simulink model "Controller1_2"  (R2018b)
settings: Solver=ode3  StartTime=0.0  StopTime=inf  FixedStep=Ts  RelTol=1e-3
InitFcn:
  | Ts=0.015; %采样时间
  | R=0.0344 %车轮半径，m
  | Wr=290 %赛道宽度290mm
  | Wc=187 %小车宽度187mm
  | Wl=250; %限宽门宽度250mm
  | K1=[0.4175;0.5498]; %速度控制的Ki、Kp参数
  | K2=[0.02;0.7]; %转向控制的Kd、Kp参数
undefined symbols (not defined in the file): DiscIntNeverNeededParam
libraries: simulink x6, legoev3lib x5, simulink_extras x1
settings Model: SimulationMode=external  ExtModeTrigDuration=2  Creator=The MathWorks, Inc.  LastModifiedBy=adminstrator
settings SolverCC: PositivePriorityOrder=on
settings DataIOCC: LimitDataPoints=on  SaveFormat=Array
settings OptimizationCC: LifeSpan=Inf  MaxStackSize=64
settings DebuggingCC: UnderspecifiedInitializationDetection=Classic  MergeDetectMultiDrivingBlocksExec=none  AllowSymbolicDim=off  SFUnexpectedBacktrackingDiag=warning  SFNoUnconditionalDefaultTransitionDiag=warning  SFExecutionAtInitializationDiag=none
settings HardwareCC: ProdBitPerPointer=32  ProdBitPerSizeT=32  ProdBitPerPtrDiffT=32  ProdLargestAtomicInteger=Long  ProdWordSize=32  ProdHWDeviceType=ARM Compatible->ARM 9  TargetLargestAtomicInteger=Long  TargetLargestAtomicFloat=Float  TargetIntDivRoundTo=Zero  TargetEndianess=LittleEndian  TargetHWDeviceType=ARM Compatible->ARM 9
settings ModelReferenceCC: PropagateSignalLabelsOutOfModel=off
settings SFSimCC: SimUseLocalCustomCode=off  SimGenImportedTypeDefs=on
settings RTWCC: SystemTargetFile=ert.tlc  HardwareBoard=LEGO MINDSTORMS EV3  TemplateMakefile=ert_default_tmf  GenerateReport=on  RTWVerbose=off  RTWUseLocalCustomCode=off  Toolchain=Sourcery G++ Lite v2009q3  BuildConfiguration=Faster Runs  LaunchReport=on
settings CodeAppCC: ForceParamTrailComments=on  OperatorAnnotations=on  StateflowObjectComments=on  MATLABSourceComments=on
settings ERTTargetCC: MultiwordLength=2048  ERTCustomFileBanners=off  SupportContinuousTime=on  SupportNonInlinedSFcns=on  RemoveResetFunc=off  ModelStepFunctionPrototypeControlCompliant=off
settings ConfigComp: CovMetricSettings=dw  CovHtmlReporting=on  CovSaveCumulativeToWorkspaceVar=on  CovSaveSingleToWorkspaceVar=on  CovExternalEMLEnable=off  CovSFcnEnable=off

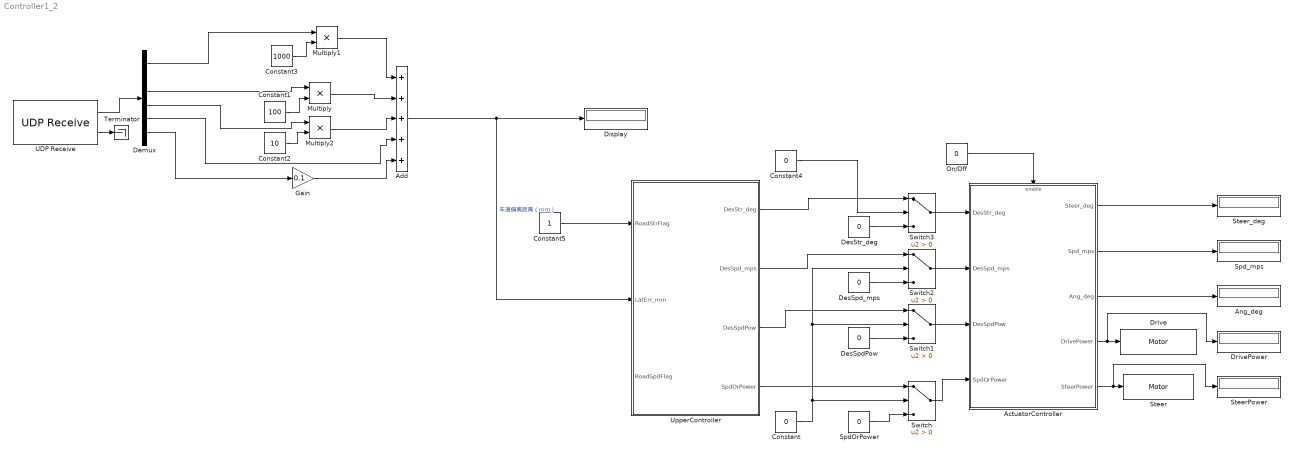
== system Controller1_2 ==
  ActuatorController : Subsystem
  Add : Sum  Inputs=+++++
  Ang_deg : Display
  Constant : Constant  Value=0
  Constant1 : Constant  Value=100
  Constant2 : Constant  Value=10
  Constant3 : Constant  Value=1000
  Constant4 : Constant  Value=0
  Constant5 : Constant
  Demux : Demux  Outputs=6
  DesSpdPow : Constant  Value=0
  DesSpd_mps : Constant  Value=0
  DesStr_deg : Constant  Value=0
  Display : Display
  Drive : legoev3lib/Motor  sportNumber=A  sstopAction=Brake
  DrivePower : Display
  Gain : Gain  Gain=0.1
  Multiply : Product
  Multiply1 : Product
  Multiply2 : Product
  On/Off : Constant  Value=0
  SpdOrPower : Constant  Value=0
  Spd_mps : Display
  Steer : legoev3lib/Motor  sportNumber=B  sstopAction=Brake
  SteerPower : Display
  Steer_deg : Display
  Switch{,1..3} (4 alike) : Switch  Criteria=u2 > Threshold
  Terminator : Terminator
  UDP Receive : legoev3lib/UDP Receive  localURL='0.0.0.0'  localPort=25000  remoteURL='0.0.0.0'  remotePort=-1  recvBufferSize=8192  signalDatatype=uint8  dims=6  isVarSize=off  showBlockingTime=off  blockingTime=0  sampletime=Ts  blockPlatform=LEGO EV3
      settings: SourceProductName=Simulink Support Package for LEGO MINDSTORMS EV3 Hardware  SourceProductBaseCode=LEGOEV3
  UpperController : Subsystem
  wires:
  On/Off/1 -> ActuatorController/Enable
  Switch/1 -> ActuatorController/4(SpdOrPower)
  Constant/1 -> Switch2/2, Switch1/2, Switch/2
  SpdOrPower/1 -> Switch/3
  DesSpdPow/1 -> Switch1/3
  Switch1/1 -> ActuatorController/3(DesSpdPow)
  Switch2/1 -> ActuatorController/2(DesSpd_mps)
  UpperController/2(DesSpd_mps) -> Switch2/1
  DesSpd_mps/1 -> Switch2/3
  Switch3/1 -> ActuatorController/1(DesStr_deg)
  Constant4/1 -> Switch3/2
  DesStr_deg/1 -> Switch3/3
  ActuatorController/5(SteerPower) -> Steer/1, SteerPower/1
  ActuatorController/1(Steer_deg) -> Steer_deg/1
  ActuatorController/2(Spd_mps) -> Spd_mps/1
  ActuatorController/3(Ang_deg) -> Ang_deg/1
  ActuatorController/4(DrivePower) -> Drive/1, DrivePower/1
  UpperController/3(DesSpdPow) -> Switch1/1
  UpperController/1(DesStr_deg) -> Switch3/1
  UpperController/4(SpdOrPower) -> Switch/1
  Demux/3 -> Multiply/1
  Constant2/1 -> Multiply2/2
  Demux/5 -> Add/4
  Multiply2/1 -> Add/3
  Multiply/1 -> Add/2
  Demux/4 -> Multiply2/1
  Add/1 -> Display/1, UpperController/2(LatErr_mm)  "车道偏离距离（mm）"
  Constant1/1 -> Multiply/2
  UDP Receive/1 -> Demux/1
  Constant3/1 -> Multiply1/2
  Multiply1/1 -> Add/1
  Demux/1 -> Multiply1/1
  UDP Receive/2 -> Terminator/1
  Constant5/1 -> UpperController/1(RoadStrFlag)
  Demux/6 -> Gain/1
  Gain/1 -> Add/5

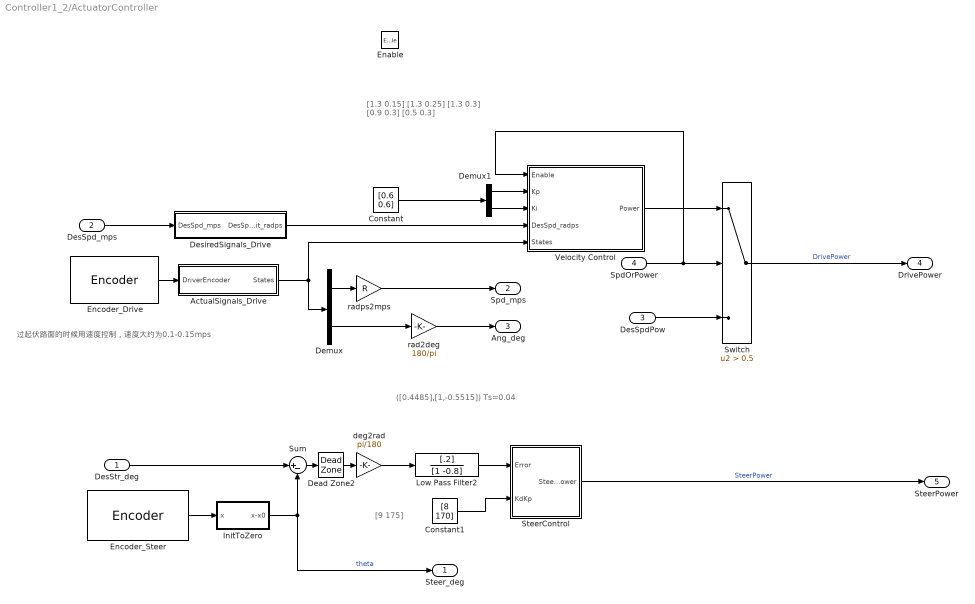
== system Controller1_2/ActuatorController ==
  note: ([0.4485],[1,-0.5515]) Ts=0.04
  note: [9 175]
  note: [1.3 0.15]
      | [1.3 0.25]
      | [1.3 0.3]
      | [0.9 0.3]
      | [0.5 0.3]
  note: 过起伏路面的时候用速度控制，速度大约为0.1-0.15mps
  DesStr_deg : Inport
  DesSpd_mps : Inport  Port=2
  DesSpdPow : Inport  Port=3
  SpdOrPower : Inport  Port=4
  Enable : EnablePort  StatesWhenEnabling=reset
  ActualSignals_Drive : Subsystem
  Constant : Constant  Value=[0.6 0.6]
  Constant1 : Constant  Value=[8 170]
  Dead Zone2 : DeadZone  LowerValue=-1  UpperValue=1  SaturateOnIntegerOverflow=on
  Demux : Demux  Outputs=2
  Demux1 : Demux  Outputs=2
  DesiredSignals_Drive : Subsystem
  Encoder_Drive : legoev3lib/Encoder  portNumber=A  opMode=No reset  sampleTime=Ts
      settings: SourceProductName=Simulink Support Package for LEGO MINDSTORMS EV3 Hardware  SourceProductBaseCode=LEGOEV3
  Encoder_Steer : legoev3lib/Encoder  portNumber=B  opMode=No reset  sampleTime=Ts
      settings: SourceProductName=Simulink Support Package for LEGO MINDSTORMS EV3 Hardware  SourceProductBaseCode=LEGOEV3
  InitToZero : Subsystem
  Low Pass Filter2 : DiscreteFilter  Numerator=[.2]  Denominator=[1 -0.8]
  SteerControl : Subsystem
  Sum : Sum  Inputs=|+-
  Switch : Switch  Criteria=u2 > Threshold  Threshold=0.5
  Velocity Control : Subsystem
  deg2rad : Gain  Gain=pi/180
  rad2deg : Gain  Gain=180/pi
  radps2mps : Gain  Gain=R
  Steer_deg : Outport
  Spd_mps : Outport  Port=2
  Ang_deg : Outport  Port=3
  DrivePower : Outport  Port=4  OutputWhenDisabled=reset  InitialOutput=0
  SteerPower : Outport  Port=5  OutputWhenDisabled=reset  InitialOutput=0
  wires:
  deg2rad/1 -> Low Pass Filter2/1
  Demux1/1 -> Velocity Control/2(Kp)
  Demux/2 -> rad2deg/1
  DesiredSignals_Drive/1(DesSpdFit_radps) -> Velocity Control/4(DesSpd_radps)
  Dead Zone2/1 -> deg2rad/1
  radps2mps/1 -> Spd_mps/1
  rad2deg/1 -> Ang_deg/1
  Demux1/2 -> Velocity Control/3(Ki)
  Constant1/1 -> SteerControl/2(KdKp)
  InitToZero/1(x-x0) -> Steer_deg/1, Sum/2  "theta"
  ActualSignals_Drive/1("States ") -> Demux/1, Velocity Control/5(States)
  SpdOrPower/1 -> Switch/2, Velocity Control/1("Enable ")
  DesStr_deg/1 -> Sum/1
  Constant/1 -> Demux1/1
  Sum/1 -> Dead Zone2/1
  Encoder_Drive/1 -> ActualSignals_Drive/1(DriverEncoder)
  Velocity Control/1(Power) -> Switch/1
  Demux/1 -> radps2mps/1
  DesSpd_mps/1 -> DesiredSignals_Drive/1(DesSpd_mps)
  Encoder_Steer/1 -> InitToZero/1(x)
  Low Pass Filter2/1 -> SteerControl/1(Error)
  Switch/1 -> DrivePower/1  "DrivePower"
  SteerControl/1(SteerPower) -> SteerPower/1  "SteerPower"
  DesSpdPow/1 -> Switch/3

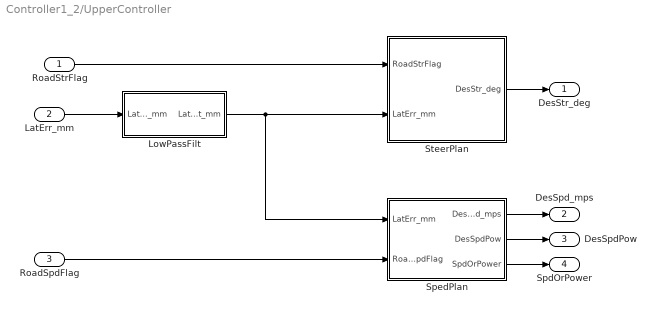
== system Controller1_2/UpperController ==
  RoadStrFlag : Inport
  LatErr_mm : Inport  Port=2
  RoadSpdFlag : Inport  Port=3
  LowPassFilt : Subsystem
  SpedPlan : Subsystem
  SteerPlan : Subsystem
  DesStr_deg : Outport
  DesSpd_mps : Outport  Port=2
  DesSpdPow : Outport  Port=3
  SpdOrPower : Outport  Port=4
  wires:
  LatErr_mm/1 -> LowPassFilt/1(LatErr_mm)
  LowPassFilt/1(LatErrFit_mm) -> SpedPlan/1(LatErr_mm), SteerPlan/2(LatErr_mm)
  SteerPlan/1(DesStr_deg) -> DesStr_deg/1
  SpedPlan/1(DesSpd_mps) -> DesSpd_mps/1
  SpedPlan/2(DesSpdPow) -> DesSpdPow/1
  SpedPlan/3(SpdOrPower) -> SpdOrPower/1
  RoadSpdFlag/1 -> SpedPlan/2(RoadSpdFlag)
  RoadStrFlag/1 -> SteerPlan/1(RoadStrFlag)

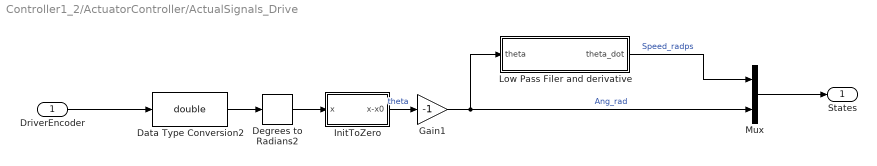
== system Controller1_2/ActuatorController/ActualSignals_Drive ==
  DriverEncoder : Inport
  Data Type Conversion2 : DataTypeConversion  OutDataTypeStr=double
  Degrees to Radians2 : simulink_extras/Transformations/Degrees to Radians
  Gain1 : Gain  Gain=-1
  InitToZero : Subsystem
  Low Pass Filer and derivative : Subsystem
  Mux : Mux  Inputs=2
  "States " : Outport
  wires:
  Degrees to Radians2/1 -> InitToZero/1(x)
  Data Type Conversion2/1 -> Degrees to Radians2/1
  InitToZero/1(x-x0) -> Gain1/1  "theta"
  DriverEncoder/1 -> Data Type Conversion2/1
  Gain1/1 -> Low Pass Filer and derivative/1(theta), Mux/2  "Ang_rad"
  Mux/1 -> "States "/1
  Low Pass Filer and derivative/1(theta_dot) -> Mux/1  "Speed_radps"

== system Controller1_2/ActuatorController/DesiredSignals_Drive ==
  DesSpd_mps : Inport
  Low Pass Filter2 : DiscreteFilter  Numerator=[0.15]  Denominator=[1 -0.85]
  m/s --> rad/s : Gain  Gain=1/R
  DesSpdFit_radps : Outport
  wires:
  m/s --> rad/s/1 -> Low Pass Filter2/1  "des_theta_dot"
  DesSpd_mps/1 -> m/s --> rad/s/1
  Low Pass Filter2/1 -> DesSpdFit_radps/1

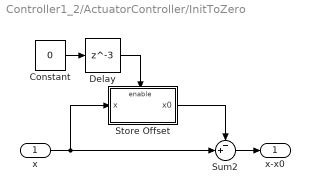
== system Controller1_2/ActuatorController/InitToZero ==
  x : Inport
  Constant : Constant  Value=0  OutDataTypeStr=boolean
  Delay : Delay  DelayLength=3  InitialCondition=1
  Store Offset : Subsystem  TreatAsAtomicUnit=on
  Sum2 : Sum  Inputs=-+|
  x-x0 : Outport
  wires:
  x/1 -> Sum2/2, Store Offset/1(x)
  Store Offset/1(x0) -> Sum2/1
  Constant/1 -> Delay/1
  Delay/1 -> Store Offset/Enable
  Sum2/1 -> x-x0/1

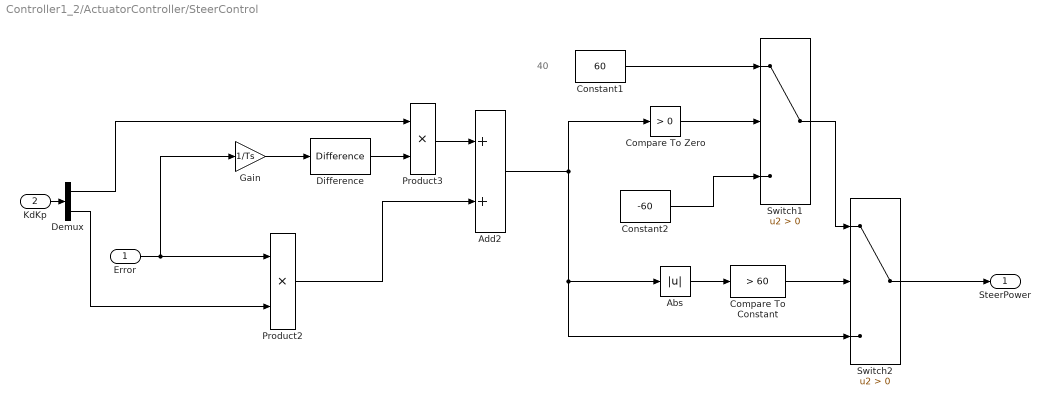
== system Controller1_2/ActuatorController/SteerControl ==
  note: 40
  Error : Inport
  KdKp : Inport  Port=2
  Abs : Abs
  Add2 : Sum
  Compare To Constant : simulink/Logic and Bit Operations/Compare To Constant  relop=>  const=60  OutDataTypeStr=boolean
  Compare To Zero : simulink/Logic and Bit Operations/Compare To Zero  relop=>  OutDataTypeStr=boolean
  Constant1 : Constant  Value=60
  Constant2 : Constant  Value=-60
  Demux : Demux  Outputs=2
  Difference : simulink/Discrete/Difference  ICPrevInput=0.0  OutMin=[]  OutMax=[]  OutDataType=fixdt(1, 16)  OutScaling=2^-10  DoSatur=off
  Gain : Gain  Gain=1/Ts
  Product2 : Product
  Product3 : Product
  Switch1 : Switch  Criteria=u2 > Threshold
  Switch2 : Switch  Criteria=u2 > Threshold
  SteerPower : Outport
  wires:
  Constant1/1 -> Switch1/1
  Switch2/1 -> SteerPower/1
  Demux/2 -> Product2/2
  Difference/1 -> Product3/2
  Add2/1 -> Compare To Zero/1, Switch2/3, Abs/1
  Product2/1 -> Add2/2
  Compare To Constant/1 -> Switch2/2
  Demux/1 -> Product3/1
  Product3/1 -> Add2/1
  Compare To Zero/1 -> Switch1/2
  Constant2/1 -> Switch1/3
  Switch1/1 -> Switch2/1
  Abs/1 -> Compare To Constant/1
  Error/1 -> Gain/1, Product2/1
  Gain/1 -> Difference/1
  KdKp/1 -> Demux/1

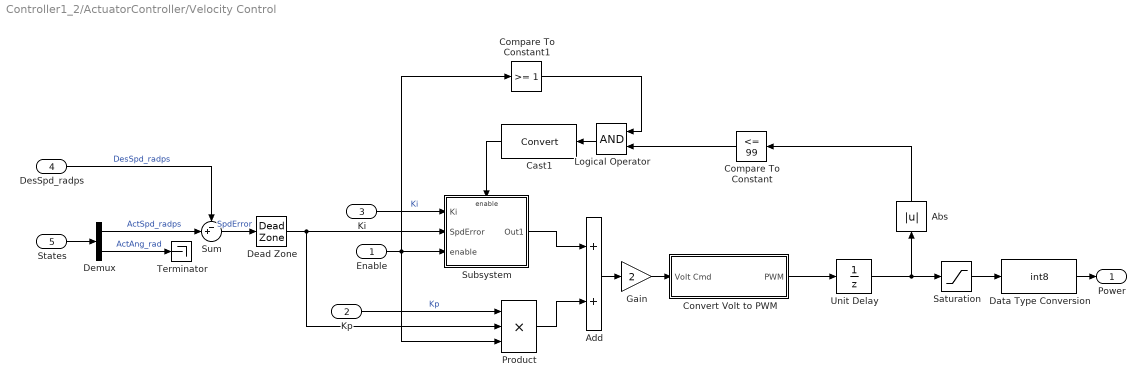
== system Controller1_2/ActuatorController/Velocity Control ==
  "Enable " : Inport
  Kp : Inport  Port=2
  Ki : Inport  Port=3
  DesSpd_radps : Inport  Port=4
  States : Inport  Port=5
  Abs : Abs
  Add : Sum
  Cast1 : DataTypeConversion
  Compare To Constant : simulink/Logic and Bit Operations/Compare To Constant  relop=<=  const=99  OutDataTypeStr=boolean
  Compare To Constant1 : simulink/Logic and Bit Operations/Compare To Constant  relop=>=  const=1  OutDataTypeStr=boolean
  Convert Volt to PWM : Subsystem
  Data Type Conversion : DataTypeConversion  OutDataTypeStr=int8
  Dead Zone : DeadZone  LowerValue=-0.01  UpperValue=0.01  SaturateOnIntegerOverflow=on
  Demux : Demux  Outputs=2
  Gain : Gain  Gain=2
  Logical Operator : Logic  AllPortsSameDT=off  OutDataTypeStr=boolean
  Product : Product  Inputs=3
  Saturation : Saturate  UpperLimit=100  LowerLimit=-100
  Subsystem : Subsystem
  Sum : Sum  Inputs=-+|
  Terminator : Terminator
  Unit Delay : UnitDelay  SampleTime=-1
  Power : Outport  OutputWhenDisabled=reset  InitialOutput=0
  wires:
  Add/1 -> Gain/1
  Gain/1 -> Convert Volt to PWM/1(Volt Cmd)
  DesSpd_radps/1 -> Sum/1  "DesSpd_radps"
  States/1 -> Demux/1
  Demux/1 -> Sum/2  "ActSpd_radps"
  Demux/2 -> Terminator/1  "ActAng_rad"
  Sum/1 -> Dead Zone/1  "SpdError"
  Ki/1 -> Subsystem/1(Ki)  "Ki"
  Product/1 -> Add/2
  Subsystem/1(Out1) -> Add/1
  Kp/1 -> Product/1  "Kp"
  Abs/1 -> Compare To Constant/1
  Compare To Constant/1 -> Logical Operator/2
  Data Type Conversion/1 -> Power/1
  Saturation/1 -> Data Type Conversion/1
  Compare To Constant1/1 -> Logical Operator/1
  Logical Operator/1 -> Cast1/1
  Cast1/1 -> Subsystem/Enable
  Convert Volt to PWM/1(PWM) -> Unit Delay/1
  "Enable "/1 -> Product/3, Compare To Constant1/1, Subsystem/3(enable)
  Unit Delay/1 -> Saturation/1, Abs/1
  Dead Zone/1 -> Product/2, Subsystem/2(SpdError)

== system Controller1_2/UpperController/LowPassFilt ==
  LatErr_mm : Inport
  Discrete Filter : DiscreteFilter  Numerator=[0.2 0.3669]  Denominator=[1 -0.4331]
  LatErrFit_mm : Outport
  wires:
  LatErr_mm/1 -> Discrete Filter/1
  Discrete Filter/1 -> LatErrFit_mm/1

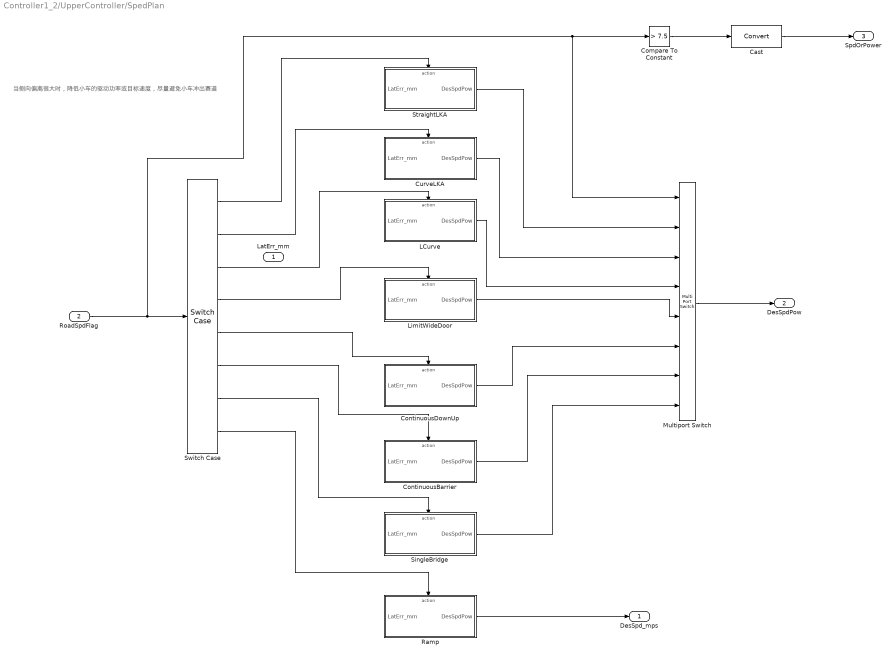
== system Controller1_2/UpperController/SpedPlan ==
  note: 当侧向偏离很大时，降低小车的驱动功率或目标速度，尽量避免小车冲出赛道
  LatErr_mm : Inport
  RoadSpdFlag : Inport  Port=2
  Cast : DataTypeConversion
  Compare To Constant : simulink/Logic and Bit Operations/Compare To Constant  relop=>  const=7.5  OutDataTypeStr=boolean
  ContinuousBarrier : Subsystem  TreatAsAtomicUnit=on
  ContinuousDownUp : Subsystem  TreatAsAtomicUnit=on
  CurveLKA : Subsystem  TreatAsAtomicUnit=on
  LCurve : Subsystem  TreatAsAtomicUnit=on
  LimitWideDoor : Subsystem  TreatAsAtomicUnit=on
  Multiport Switch : MultiPortSwitch  Inputs=7
  Ramp : Subsystem  TreatAsAtomicUnit=on
  SingleBridge : Subsystem  TreatAsAtomicUnit=on
  StraightLKA : Subsystem  TreatAsAtomicUnit=on
  Switch Case : SwitchCase  CaseConditions={1,2,3,4,5,6,7,8}  ShowDefaultCase=off
  DesSpd_mps : Outport
  DesSpdPow : Outport  Port=2
  SpdOrPower : Outport  Port=3
  wires:
  Switch Case/1 -> StraightLKA/Action
  Switch Case/2 -> CurveLKA/Action
  Switch Case/3 -> LCurve/Action
  Switch Case/4 -> LimitWideDoor/Action
  Switch Case/5 -> ContinuousDownUp/Action
  Switch Case/6 -> ContinuousBarrier/Action
  Switch Case/7 -> SingleBridge/Action
  Switch Case/8 -> Ramp/Action
  Multiport Switch/1 -> DesSpdPow/1
  RoadSpdFlag/1 -> Multiport Switch/1, Compare To Constant/1, Switch Case/1
  StraightLKA/1(DesSpdPow) -> Multiport Switch/2
  CurveLKA/1(DesSpdPow) -> Multiport Switch/3
  LCurve/1(DesSpdPow) -> Multiport Switch/4
  LimitWideDoor/1(DesSpdPow) -> Multiport Switch/5
  ContinuousDownUp/1(DesSpdPow) -> Multiport Switch/6
  ContinuousBarrier/1(DesSpdPow) -> Multiport Switch/7
  SingleBridge/1(DesSpdPow) -> Multiport Switch/8
  Ramp/1(DesSpdPow) -> DesSpd_mps/1
  Compare To Constant/1 -> Cast/1
  Cast/1 -> SpdOrPower/1

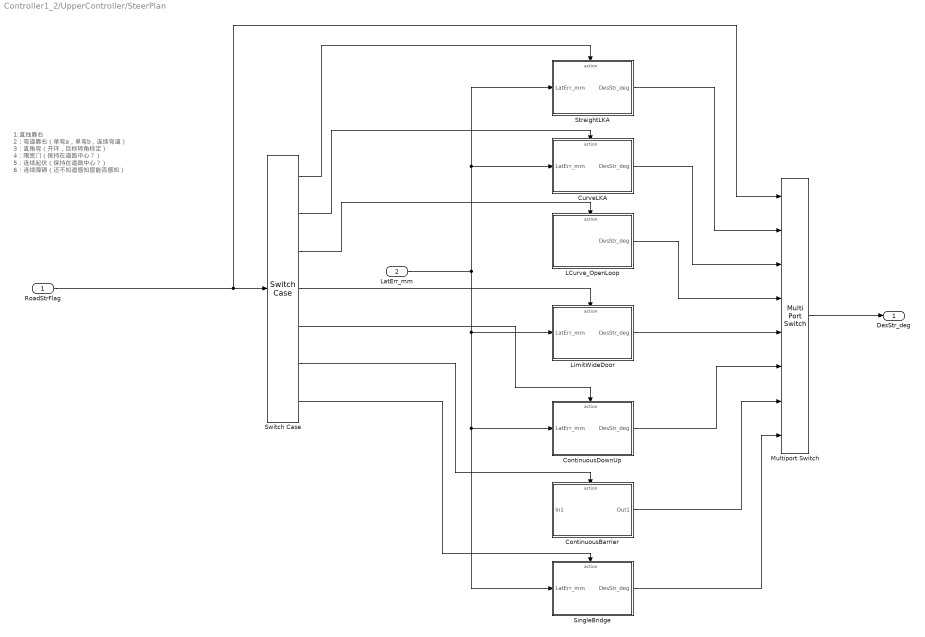
== system Controller1_2/UpperController/SteerPlan ==
  note: 1:直线靠右
      | 2：弯道靠右（单弯a，单弯b，连续弯道）
      | 3：直角弯（开环，目标转角标定）
      | 4：限宽门（保持在道路中心？）
      | 5：连续起伏（保持在道路中心？）
      | 6：连续障碍（还不知道感知层能否感知）
  RoadStrFlag : Inport
  LatErr_mm : Inport  Port=2
  ContinuousBarrier : Subsystem  TreatAsAtomicUnit=on
  ContinuousDownUp : Subsystem  TreatAsAtomicUnit=on
  CurveLKA : Subsystem  TreatAsAtomicUnit=on
  LCurve_OpenLoop : Subsystem  TreatAsAtomicUnit=on
  LimitWideDoor : Subsystem  TreatAsAtomicUnit=on
  Multiport Switch : MultiPortSwitch  Inputs=7
  SingleBridge : Subsystem  TreatAsAtomicUnit=on
  StraightLKA : Subsystem  TreatAsAtomicUnit=on
  Switch Case : SwitchCase  CaseConditions={1,2,3,4,5,6,7}  ShowDefaultCase=off
  DesStr_deg : Outport
  wires:
  RoadStrFlag/1 -> Multiport Switch/1, Switch Case/1
  Switch Case/2 -> CurveLKA/Action
  Switch Case/3 -> LCurve_OpenLoop/Action
  Switch Case/4 -> LimitWideDoor/Action
  Switch Case/5 -> ContinuousDownUp/Action
  Switch Case/6 -> ContinuousBarrier/Action
  Multiport Switch/1 -> DesStr_deg/1
  StraightLKA/1(DesStr_deg) -> Multiport Switch/2
  CurveLKA/1(DesStr_deg) -> Multiport Switch/3
  LCurve_OpenLoop/1(DesStr_deg) -> Multiport Switch/4
  LimitWideDoor/1(DesStr_deg) -> Multiport Switch/5
  ContinuousDownUp/1(DesStr_deg) -> Multiport Switch/6
  ContinuousBarrier/1(Out1) -> Multiport Switch/7
  LatErr_mm/1 -> CurveLKA/1(LatErr_mm), StraightLKA/1(LatErr_mm), LimitWideDoor/1(LatErr_mm), SingleBridge/1(LatErr_mm), ContinuousDownUp/1(LatErr_mm)
  Switch Case/7 -> SingleBridge/Action
  Switch Case/1 -> StraightLKA/Action
  SingleBridge/1(DesStr_deg) -> Multiport Switch/8

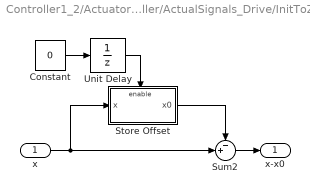
== system Controller1_2/ActuatorController/ActualSignals_Drive/InitToZero ==
  x : Inport
  Constant : Constant  Value=0  OutDataTypeStr=boolean
  Store Offset : Subsystem  TreatAsAtomicUnit=on
  Sum2 : Sum  Inputs=-+|
  Unit Delay : UnitDelay  InitialCondition=1  SampleTime=-1
  x-x0 : Outport
  wires:
  x/1 -> Sum2/2, Store Offset/1(x)
  Store Offset/1(x0) -> Sum2/1
  Constant/1 -> Unit Delay/1
  Unit Delay/1 -> Store Offset/Enable
  Sum2/1 -> x-x0/1

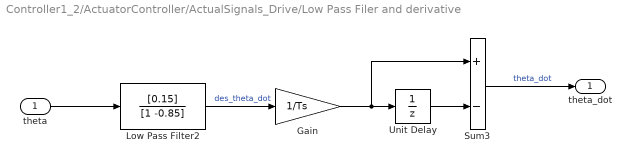
== system Controller1_2/ActuatorController/ActualSignals_Drive/Low Pass Filer and derivative ==
  theta : Inport
  Gain : Gain  Gain=1/Ts
  Low Pass Filter2 : DiscreteFilter  Numerator=[0.15]  Denominator=[1 -0.85]
  Sum3 : Sum  Inputs=+-
  Unit Delay : UnitDelay  SampleTime=-1
  theta_dot : Outport
  wires:
  theta/1 -> Low Pass Filter2/1
  Sum3/1 -> theta_dot/1  "theta_dot"
  Gain/1 -> Sum3/1, Unit Delay/1
  Unit Delay/1 -> Sum3/2
  Low Pass Filter2/1 -> Gain/1  "des_theta_dot"

== system Controller1_2/ActuatorController/InitToZero/Store Offset ==
  x : Inport
  Enable : EnablePort
  x0 : Outport  InitialOutput=0
  wires:
  x/1 -> x0/1

== system Controller1_2/ActuatorController/Velocity Control/Convert Volt to PWM ==
  note: Normalization by maximum voltage
      | and
      | Scaling to PWM
  Volt Cmd : Inport
  Battery Voltage : Subsystem
  Divide : Product  Inputs=*/
  Gain : Gain  Gain=100
  Low Pass Filter : DiscreteFilter  Numerator=[0.15]  Denominator=[1 -0.85]
  PWM : Outport
  wires:
  Battery Voltage/1(Battery) -> Divide/2
  Divide/1 -> Gain/1
  Volt Cmd/1 -> Low Pass Filter/1  "des_theta_dot"
  Gain/1 -> PWM/1
  Low Pass Filter/1 -> Divide/1

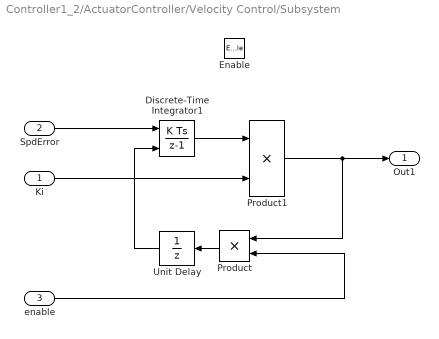
== system Controller1_2/ActuatorController/Velocity Control/Subsystem ==
  Ki : Inport
  SpdError : Inport  Port=2
  enable : Inport  Port=3
  Enable : EnablePort  StatesWhenEnabling=reset
  Discrete-Time Integrator1 : DiscreteIntegrator  InitialConditionSource=external  SampleTime=-1  ICPrevOutput=DiscIntNeverNeededParam  ICPrevScaledInput=DiscIntNeverNeededParam
  Product : Product
  Product1 : Product
  Unit Delay : UnitDelay  SampleTime=-1
  Out1 : Outport
  wires:
  Ki/1 -> Product1/2
  Discrete-Time Integrator1/1 -> Product1/1
  Product1/1 -> Product/1, Out1/1
  SpdError/1 -> Discrete-Time Integrator1/1
  enable/1 -> Product/2
  Product/1 -> Unit Delay/1
  Unit Delay/1 -> Discrete-Time Integrator1/2

== system Controller1_2/UpperController/SpedPlan/ContinuousBarrier ==
  LatErr_mm : Inport
  Action Port : ActionPort  ActionType=case
  DesSpdPow : Outport
  wires:
  LatErr_mm/1 -> DesSpdPow/1

== system Controller1_2/UpperController/SpedPlan/ContinuousDownUp ==
  LatErr_mm : Inport
  Action Port : ActionPort  ActionType=case
  DesSpdPow : Outport
  wires:
  LatErr_mm/1 -> DesSpdPow/1

== system Controller1_2/UpperController/SpedPlan/CurveLKA ==
  LatErr_mm : Inport
  Action Port : ActionPort  ActionType=case
  DesSpdPow : Outport
  wires:
  LatErr_mm/1 -> DesSpdPow/1

== system Controller1_2/UpperController/SpedPlan/LCurve ==
  LatErr_mm : Inport
  Action Port : ActionPort  ActionType=case
  DesSpdPow : Outport
  wires:
  LatErr_mm/1 -> DesSpdPow/1

== system Controller1_2/UpperController/SpedPlan/LimitWideDoor ==
  LatErr_mm : Inport
  Action Port : ActionPort  ActionType=case
  DesSpdPow : Outport
  wires:
  LatErr_mm/1 -> DesSpdPow/1

== system Controller1_2/UpperController/SpedPlan/Ramp ==
  LatErr_mm : Inport
  Action Port : ActionPort  ActionType=case
  DesSpdPow : Outport
  wires:
  LatErr_mm/1 -> DesSpdPow/1

== system Controller1_2/UpperController/SpedPlan/SingleBridge ==
  LatErr_mm : Inport
  Action Port : ActionPort  ActionType=case
  DesSpdPow : Outport
  wires:
  LatErr_mm/1 -> DesSpdPow/1

== system Controller1_2/UpperController/SpedPlan/StraightLKA ==
  LatErr_mm : Inport
  Action Port : ActionPort  ActionType=case
  DesSpdPow : Outport
  wires:
  LatErr_mm/1 -> DesSpdPow/1

== system Controller1_2/UpperController/SteerPlan/ContinuousBarrier ==
  In1 : Inport
  Action Port : ActionPort  ActionType=case
  Out1 : Outport
  wires:
  In1/1 -> Out1/1

== system Controller1_2/UpperController/SteerPlan/ContinuousDownUp ==
  note: 和直线车道保持一样，之所以和直线LKA分开，是考虑到后续调参的时候可能会和直线LKA不太一样
  LatErr_mm : Inport
  Action Port : ActionPort  ActionType=case
  Constant : Constant  Value=Wc
  MATLAB Function : MATLAB Function  TreatAsAtomicUnit=on
  DesStr_deg : Outport
  wires:
  MATLAB Function/1(deg) -> DesStr_deg/1
  LatErr_mm/1 -> MATLAB Function/1(err)
  Constant/1 -> MATLAB Function/2(Wc)

== system Controller1_2/UpperController/SteerPlan/CurveLKA ==
  note: 和直线相比，把原来为0的位置用正负15deg代替，其他的
      | 换成正负30deg、正负45deg和正负60deg。
  LatErr_mm : Inport
  Action Port : ActionPort  ActionType=case
  Constant : Constant  Value=Wc
  Constant1 : Constant  Value=Wr
  MATLAB Function : MATLAB Function  TreatAsAtomicUnit=on
  DesStr_deg : Outport
  wires:
  MATLAB Function/1(deg) -> DesStr_deg/1
  LatErr_mm/1 -> MATLAB Function/1(err)
  Constant/1 -> MATLAB Function/2(Wc)
  Constant1/1 -> MATLAB Function/3(Wr)

== system Controller1_2/UpperController/SteerPlan/LCurve_OpenLoop ==
  Action Port : ActionPort  ActionType=case
  Constant : Constant  Value=50
  DesStr_deg : Outport
  wires:
  Constant/1 -> DesStr_deg/1

== system Controller1_2/UpperController/SteerPlan/LimitWideDoor ==
  note: 分三个等级，0，正负10deg，正负20deg，正负30deg，正负45deg，其中正负45deg主要用于
      | 从上一个工况切换到该工况时小车能快速从右侧车道切到道路中心
  LatErr_mm : Inport
  Action Port : ActionPort  ActionType=case
  Constant : Constant  Value=Wl
  Constant1 : Constant  Value=Wc
  MATLAB Function : MATLAB Function  TreatAsAtomicUnit=on
  DesStr_deg : Outport
  wires:
  LatErr_mm/1 -> MATLAB Function/1(err)
  MATLAB Function/1(deg) -> DesStr_deg/1
  Constant/1 -> MATLAB Function/3(Wl)
  Constant1/1 -> MATLAB Function/2(Wc)

== system Controller1_2/UpperController/SteerPlan/SingleBridge ==
  note: 和直线LKA的类似，只是把正负15deg、正负30deg、正负45deg改为
      | 正负10deg、正负20deg、正负30deg
  LatErr_mm : Inport
  Action Port : ActionPort  ActionType=case
  Constant : Constant  Value=Wc
  MATLAB Function : MATLAB Function  TreatAsAtomicUnit=on
  DesStr_deg : Outport
  wires:
  MATLAB Function/1(deg) -> DesStr_deg/1
  LatErr_mm/1 -> MATLAB Function/1(err)
  Constant/1 -> MATLAB Function/2(Wc)

== system Controller1_2/UpperController/SteerPlan/StraightLKA ==
  note: 1、左右各三个档，0，正负15deg、正负30deg、正负45deg
      | 往右转向为正，往左转为负
      | 2、左右各三个档，0，正负10deg、正负20deg、正负30deg
      | 往右转向为正，往左转为负
  LatErr_mm : Inport
  Action Port : ActionPort  ActionType=case
  Constant1 : Constant  Value=Wc
  Function1 : MATLAB Function  TreatAsAtomicUnit=on
  DesStr_deg : Outport
  wires:
  LatErr_mm/1 -> Function1/1(err)
  Function1/1(deg) -> DesStr_deg/1
  Constant1/1 -> Function1/2(Wc)

== system Controller1_2/ActuatorController/ActualSignals_Drive/InitToZero/Store Offset ==
  x : Inport
  Enable : EnablePort
  x0 : Outport  InitialOutput=0
  wires:
  x/1 -> x0/1

== system Controller1_2/ActuatorController/Velocity Control/Convert Volt to PWM/Battery Voltage ==
  Battery Voltage : Constant  Value=8000
  Constant : Constant  Value=0.625
  Gain1 : Gain  Gain=0.001089
  Sum : Sum  Inputs=|+-
  Battery : Outport
  wires:
  Gain1/1 -> Sum/1
  Constant/1 -> Sum/2
  Battery Voltage/1 -> Gain1/1
  Sum/1 -> Battery/1

== matlab function Controller1_2/UpperController/SteerPlan/CurveLKA/MATLAB Function ==
  data: err input; deg output; Wc input; Wr input
function deg = FcnSteer(err,Wc,Wr)
deg=0;
if err>Wc/2+44.1 && err<=Wr
    deg=15;
    return;
elseif err>=Wr && err<=Wc/2+58.8
    deg=-15;
    return;
elseif err>=Wc/2+29.4 && err<=Wc/2+44.1
    deg=30;
    return;
elseif err>=Wc/2+14.7 && err<=Wc/2+29.4
    deg=45;
    return;
elseif err<=Wc/2+14.7
    deg=60;
    return;
elseif err>=Wc/2+58.8 && err<=Wc/2+73.5
    deg=-30;
    return;
elseif err>Wc/2+73.5 && err<=Wc/2+88.2
    deg=-45;
    return;
elseif err>=Wc/2+88.2
    deg=-60;
    return;
end
end

== matlab function Controller1_2/UpperController/SteerPlan/StraightLKA/Function1 ==
  data: err input; deg output; Wc input
function deg = FcnSteer(err,Wc)
deg=0;
if err>=Wc/2+44.1 && err<=Wc/2+58.8
    deg=0;
    return;
elseif err>=Wc/2+29.4 && err<=Wc/2+44.1
    deg=15;
    return;
elseif err>=Wc/2+14.7 && err<=Wc/2+29.4
    deg=30;
    return;
elseif err<=Wc/2+14.7
    deg=45;
    return;
elseif err>=Wc/2+58.8 && err<=Wc/2+73.5
    deg=-15;
    return;
elseif err>Wc/2+73.5 && err<=Wc/2+88.2
    deg=-30;
    return;
elseif err>=Wc/2+88.2
    deg=-45;
    return;
end

== matlab function Controller1_2/UpperController/SteerPlan/ContinuousDownUp/MATLAB Function ==
  data: err input; deg output; Wc input
function deg = FcnSteer(err,Wc)
deg=0;
if err>Wc/2+44.1 && err<=Wc/2+58.8
    deg=0;
    return;
elseif err>Wc/2+29.4 && err<=Wc/2+44.1
    deg=15;
    return;
elseif err>Wc/2+14.7 && err<=Wc/2+29.4
    deg=30;
    return;
elseif err<=Wc/2+14.7
    deg=45;
    return;
elseif err>Wc/2+58.8 && err<=Wc/2+73.5
    deg=-15;
    return;
elseif err>Wc/2+73.5 && err<=Wc/2+88.2
    deg=-30;
    return;
elseif err>Wc/2+88.2
    deg=-45;
    return;
end

== matlab function Controller1_2/UpperController/SteerPlan/LimitWideDoor/MATLAB Function ==
  data: err input; deg output; Wc input; Wl input
function deg = FcnSteer(err,Wc,Wl)
deg=0;
if err>=-(Wl-Wc)/2/7 && err<=(Wl-Wc)/2/7
    deg=0;
    return;
elseif err>=-(Wl-Wc)/2/7*3 && err<=-(Wl-Wc)/2/7
    deg=10;
    return;
elseif err>=-(Wl-Wc)/2/7*5 && err<=-(Wl-Wc)/2/7*3
    deg=20;
    return;
elseif err>=-(Wl-Wc)/2/7*7 err<=-(Wl-Wc)/2/7*5
    deg=30;
    return;
elseif err<=-(Wl-Wc)/2/7*7 
    deg=45;
    return;  
elseif err>=(Wl-Wc)/2/7 && err<=(Wl-Wc)/2/7*3
    deg=-10;
    return;
elseif err>=(Wl-Wc)/2/7*3 && err<=(Wl-Wc)/2/7*5
    deg=20;
    return;
elseif err>=(Wl-Wc)/2/7*5 && err<=(Wl-Wc)/2/7*7
    deg=30;
    return;
elseif err>=(Wl-Wc)/2/7*7
    deg=45;
    return;
end

== matlab function Controller1_2/UpperController/SteerPlan/SingleBridge/MATLAB Function ==
  data: err input; deg output; Wc input
function deg = FcnSteer(err,Wc)
deg=0;
if err>Wc/2+44.1 && err<=Wc/2+58.8
    deg=0;
    return;
elseif err>Wc/2+29.4 && err<=Wc/2+44.1
    deg=10;
    return;
elseif err>Wc/2+14.7 && err<=Wc/2+29.4
    deg=20;
    return;
elseif err<=Wc/2+14.7
    deg=30;
    return;
elseif err>Wc/2+58.8 && err<=Wc/2+73.5
    deg=-10;
    return;
elseif err>Wc/2+73.5 && err<=Wc/2+88.2
    deg=-20;
    return;
elseif err>Wc/2+88.2
    deg=-30;
    return;
end
